simulink model "exa3"  (R2024a)
settings: Solver=VariableStepAuto  StartTime=0.0  StopTime=10.0  RelTol=1e-3
libraries: slpidlib x1
settings Model: Creator=Mateo  LastModifiedBy=Mateo

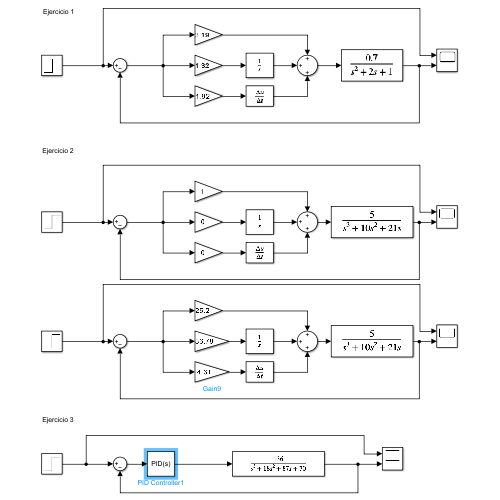
[thumbnail: Simulink's stored preview of the top-level diagram]
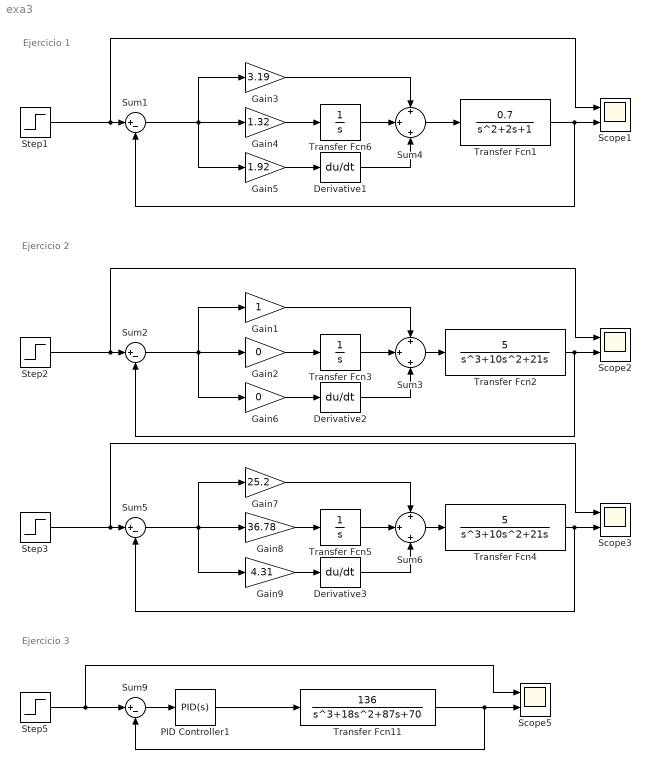
== system exa3 ==
  note: Ejercicio 2
  note: Ejercicio 3
  note: Ejercicio 1
  Derivative1 : Derivative
  Derivative2 : Derivative
  Derivative3 : Derivative
  Gain1 : Gain
  Gain2 : Gain  Gain=0
  Gain3 : Gain  Gain=3.19
  Gain4 : Gain  Gain=1.32
  Gain5 : Gain  Gain=1.92
  Gain6 : Gain  Gain=0
  Gain7 : Gain  Gain=25.2
  Gain8 : Gain  Gain=36.78
  Gain9 : Gain  Gain=4.31
  PID Controller1 : slpidlib/PID Controller  Controller=PID  Form=Parallel  TimeDomain=Continuous-time  UseExternalTs=off  SampleTime=-1  IntegratorMethod=Forward Euler  FilterMethod=Forward Euler  ControllerParametersSource=internal  P=5.37669303496244  I=5.91949026364569  UseKiTs=off  D=1.14379728369726  UseExternalDerivativeSource=off  N=1099.43284945055  UseFilter=on  TunerSelectOption=Transfer Function Based (PID Tuner App)  InitialConditionSource=internal  InitialConditionForIntegrator=0  InitialConditionForFilter=0  DifferentiatorICPrevScaledInput=0  ExternalReset=none  TrackingMode=off  Kt=1  LimitOutput=off  SatLimitsSource=internal  UpperSaturationLimit=inf  LowerSaturationLimit=-inf  LinearizeAsGain=on  AntiWindupMode=none  Kb=1  LimitIntegrator=off  UpperIntegratorSaturationLimit=inf  LowerIntegratorSaturationLimit=-inf  POutMin=[]  POutMax=[]  IOutMin=[]  IOutMax=[]  DOutMin=[]  DOutMax=[]  NOutMin=[]  NOutMax=[]  SumOutMin=[]  SumOutMax=[]  SaturationOutMin=[]  SaturationOutMax=[]  PParamMin=[]  PParamMax=[]  IParamMin=[]  IParamMax=[]  DParamMin=[]  DParamMax=[]  NParamMin=[]  NParamMax=[]  KbParamMin=[]  KbParamMax=[]  KtParamMin=[]  KtParamMax=[]  KbOutMin=[]  KbOutMax=[]  KtOutMin=[]  KtOutMax=[]  IntegratorOutMin=[]  IntegratorOutMax=[]  FilterOutMin=[]  FilterOutMax=[]  SumI1OutMin=[]  SumI1OutMax=[]  SumI2OutMin=[]  SumI2OutMax=[]  SumI3OutMin=[]  SumI3OutMax=[]  SumI4OutMin=[]  SumI4OutMax=[]  SumDOutMin=[]  SumDOutMax=[]  DifferentiatorOutMin=[]  DifferentiatorOutMax=[]  FilterDiffOutCoefMin=[]  FilterDiffOutCoefMax=[]  ReciprocalOutMin=[]  ReciprocalOutMax=[]  SumDenOutMin=[]  SumDenOutMax=[]  SumNumOutMin=[]  SumNumOutMax=[]  DivideOutMin=[]  DivideOutMax=[]  UdiffTsProdOutMin=[]  UdiffTsProdOutMax=[]  NTsProdOutMin=[]  NTsProdOutMax=[]  UintegralTsProdOutMin=[]  UintegralTsProdOutMax=[]  UngainTsProdOutMin=[]  UngainTsProdOutMax=[]  ClampingZeroOutDataTypeStr=Inherit: Inherit via back propagation  ClampingZeroOutMin=[]  ClampingZeroOutMax=[]  FilterDenConstantOutDataTypeStr=Inherit: Inherit via back propagation  FilterDenConstantOutMin=[]  FilterDenConstantOutMax=[]  PCopyOutDataTypeStr=Inherit: Inherit via back propagation  PCopyOutMin=[]  PCopyOutMax=[]  NCopyOutDataTypeStr=Inherit: Inherit via back propagation  NCopyOutMin=[]  NCopyOutMax=[]  IntegratorContinuousStateAttributes=''  IntegratorStateMustResolveToSignalObject=off  IntegratorRTWStateStorageClass=Auto  FilterContinuousStateAttributes=''  FilterStateMustResolveToSignalObject=off  FilterRTWStateStorageClass=Auto  ParallelPVariant=InternalParameters  IdealPVariant=Disabled  IVariant=InternalParameters  DVariant=InternalParameters  IntegratorVariant=Continuous  SatVariant=Disabled  AWVariant=Passthrough  PCopyVariant=Disabled  TRVariant=Disabled  FdbkBlocksVariant=Forward  IdealPFdbkVariant=Disabled  SatFdbkVariant=Disabled  DerivativeFilterVariant=ContFilter  NVariant=InternalParameters  NCopyVariant=Disabled  FilterICVariant=InternalICsFilter  IntegratorICVariant=InternalICs  ExternalResetVariant=Disabled  TRSumVariant=Passthrough  SumFdbkVariant=Disabled  SumVariant=Sum_PID  TsampFilterVariant=InternalTs  TsampNgainVariant=Passthrough  TsampIntegralVariant=Disabled_SignalSpec  ExternalSaturationOutDataTypeStr=Inherit: Same as second input  DerivativeSourceVariant=ErrorSignal
  Scope{1..3,5} (4 alike) : Scope  NumInputPorts=2
  Step{1..3,5} (4 alike) : Step  SampleTime=0
  Sum{1..2,5,9} (4 alike) : Sum  Inputs=|+-
  Sum3 : Sum  Inputs=+|+|+
  Sum4 : Sum  Inputs=+|+|+
  Sum6 : Sum  Inputs=+|+|+
  Transfer Fcn1 : TransferFcn  Numerator=0.7
  Transfer Fcn11 : TransferFcn  Numerator=[136]  Denominator=[1 18 87 70]
  Transfer Fcn2 : TransferFcn  Numerator=5  Denominator=[1 10 21 0]
  Transfer Fcn3 : TransferFcn  Denominator=[1 0]
  Transfer Fcn4 : TransferFcn  Numerator=5  Denominator=[1 10 21 0]
  Transfer Fcn5 : TransferFcn  Denominator=[1 0]
  Transfer Fcn6 : TransferFcn  Denominator=[1 0]
  wires:
  Transfer Fcn6/1 -> Sum4/2
  PID Controller1/1 -> Transfer Fcn11/1
  Transfer Fcn11/1 -> Sum9/2, Scope5/2
  Step5/1 -> Scope5/1, Sum9/1
  Step1/1 -> Sum1/1, Scope1/1
  Gain3/1 -> Sum4/1
  Sum1/1 -> Gain3/1, Gain4/1, Gain5/1
  Derivative1/1 -> Sum4/3
  Gain5/1 -> Derivative1/1
  Gain4/1 -> Transfer Fcn6/1
  Sum4/1 -> Transfer Fcn1/1
  Transfer Fcn1/1 -> Scope1/2, Sum1/2
  Sum9/1 -> PID Controller1/1
  Transfer Fcn2/1 -> Scope2/2, Sum2/2
  Gain2/1 -> Transfer Fcn3/1
  Sum3/1 -> Transfer Fcn2/1
  Sum2/1 -> Gain1/1, Gain2/1, Gain6/1
  Gain6/1 -> Derivative2/1
  Derivative2/1 -> Sum3/3
  Transfer Fcn3/1 -> Sum3/2
  Gain1/1 -> Sum3/1
  Step2/1 -> Sum2/1, Scope2/1
  Gain7/1 -> Sum6/1
  Step3/1 -> Sum5/1, Scope3/1
  Transfer Fcn5/1 -> Sum6/2
  Derivative3/1 -> Sum6/3
  Gain9/1 -> Derivative3/1
  Sum6/1 -> Transfer Fcn4/1
  Gain8/1 -> Transfer Fcn5/1
  Sum5/1 -> Gain7/1, Gain8/1, Gain9/1
  Transfer Fcn4/1 -> Scope3/2, Sum5/2
